simulink model "DSB"  (R2014b)
settings: Solver=ode45  StartTime=0.0  StopTime=10.0  RelTol=1e-3
libraries: dsparch4 x1, commnoisgen2 x1
settings Model: Creator=TY  LastModifiedBy=TY

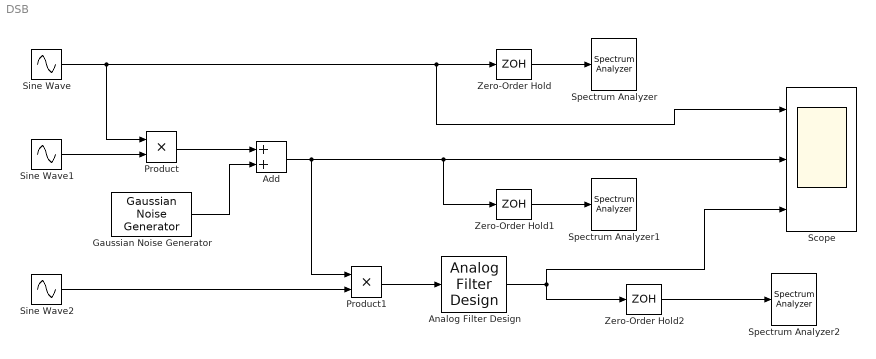
== system DSB ==
  Add : Sum
  Analog Filter Design : dsparch4/Analog Filter Design  method=Butterworth  filttype=Lowpass  N=8  Wlo=25*6.28  Whi=80  Rp=2  Rs=40
  Gaussian Noise Generator : commnoisgen2/Gaussian Noise Generator  m=0  d=0.01  s=41  Ts=1/1000  frameBased=off  sampPerFrame=1  orient=off  outDataType=double
  Product : Product
  Product1 : Product
  Scope : Scope  NumInputPorts=3
      settings: TimeRange=1.59968  YMin=-5~-1~-5  YMax=5~1~5
  Sine Wave : Sin  Frequency=20*6.28  SampleTime=0
  Sine Wave1 : Sin  Frequency=200*6.28  SampleTime=0
  Sine Wave2 : Sin  Amplitude=2  Frequency=200*6.28  SampleTime=0
  Spectrum Analyzer : SpectrumAnalyzer
  Spectrum Analyzer1 : SpectrumAnalyzer
  Spectrum Analyzer2 : SpectrumAnalyzer
  Zero-Order Hold : ZeroOrderHold  SampleTime=1/1000
  Zero-Order Hold1 : ZeroOrderHold  SampleTime=1/10000
  Zero-Order Hold2 : ZeroOrderHold  SampleTime=1/1000
  wires:
  Sine Wave/1 -> Product/1, Scope/1, Zero-Order Hold/1
  Sine Wave1/1 -> Product/2
  Sine Wave2/1 -> Product1/2
  Product1/1 -> Analog Filter Design/1
  Zero-Order Hold/1 -> Spectrum Analyzer/1
  Zero-Order Hold1/1 -> Spectrum Analyzer1/1
  Analog Filter Design/1 -> Scope/3, Zero-Order Hold2/1
  Zero-Order Hold2/1 -> Spectrum Analyzer2/1
  Product/1 -> Add/1
  Gaussian Noise Generator/1 -> Add/2
  Add/1 -> Product1/1, Zero-Order Hold1/1, Scope/2
